simulink model "HighClearance_model"  (R2019b)
settings: configuration reference "configRef" (kept outside this file)
undefined symbols (not defined in the file): baseClearance, calSTEP1_e, calSTEP2_e, calSTEP3_e, calSTEP4_e, calTolMultiplier, errorMinSpd, heightCalibrating_e, heightDiffTolerance, heightDown_e, heightError_e, heightMovingDown_e, heightMovingUp_e, heightUnknown_e, heightUp_e, IOD_OK, IOD_Open, IOD_ScGnd, maxMedianWheelAngle, maxTransitionMachineSpd, minTransitionMachineSpd, positionSensor_tblData, positionSensorFL_BrkPnts, positionSensorFR_BrkPnts, positionSensorRL_BrkPnts, positionSensorRR_BrkPnts, step_time, trackWidthMax, trackWidthMin, trackWidthTolerance, twoWheelSteer
libraries: HighClearance_library x129, simulink x25
(part 3 of 3)

== stateflow chart HighClearance_model/Arbitration/TargetStateArbitration ==
  state states
    en,du: lowerOkay = ( okayToLower() && !disableLower() );
    raiseOkay = ( okayToRaise() && !disableRiase() );
    state out = leaveActiveState [function]
      (default) -> (junction 1676)
      (junction 1685) -> (junction 1686) [order 1] : [prevTargetState == heightMovingDown_e]
      (junction 1676) -> (junction 1685) [order 1] : [hasChangedTo(stopBtn,1)]
      (junction 1676) -> (junction 1696) [order 2]
      (junction 1685) -> (junction 1687) [order 2]
      (junction 1686) -> (junction 1690)
      (junction 1687) -> (junction 1690) : [prevTargetState == heightMovingUp_e]
      (junction 1690) -> (junction 1698)
      (junction 1696) -> (junction 1698) [order 1] : [manualOverride != 0]
      (junction 1696) -> (junction 1701) [order 2]
      (junction 1698) -> (junction 1700)
      (junction 1701) -> (junction 1700) [order 1] : [!calOkay()]
      (junction 1701) -> (junction 1711) [order 2]
      (junction 1700) -> (junction 1712)
      (junction 1711) -> (junction 1705) [order 1] : [prevTargetState == heightMovingDown_e]
      (junction 1705) -> (junction 1712) : [disableLower()]
      (junction 1711) -> (junction 1713) [order 2]
      (junction 1712) -> (junction 1714)
      (junction 1713) -> (junction 1706) [order 1] : [prevTargetState == heightMovingUp_e]
      (junction 1706) -> (junction 1714) : [disableRiase()]
      (junction 1713) -> (junction 1716) [order 2]
      (junction 1714) -> (junction 1717)
      (junction 1716) -> (junction 1717) [order 1] : [noMovementErr()]
      (junction 1716) -> (junction 1742) [order 2]
      (junction 1717) -> (junction 1734)
      (junction 1742) -> (junction 1733) [order 1] : [hasChangedTo(downBtn,1)]
      (junction 1733) -> (junction 1734) : [targetStateDown()]
      (junction 1742) -> (junction 1744) [order 2]
      (junction 1734) -> (junction 1738)
      (junction 1737) -> (junction 1738) : [targetStateUp()]
      (junction 1744) -> (junction 1737) [order 1] : [hasChangedTo(upBtn,1)]
      (junction 1744) -> (junction 1725) [order 2]
      (junction 1738) -> (junction 1728)
      (junction 1728) -> (junction 1730) : {out = true}
      (junction 1730) -> (junction 1723)
      (junction 1725) -> (junction 1723) : {out = false}
    state clearWarnings [function]
      (default) -> (junction 687) : {activeWarnings.trackWidth = 0;
          | activeWarnings.speed = 0;
          | activeWarnings.guide = 0;
          | activeWarnings.was = 0;
          | activeWarnings.fws = 0;
          | activeWarnings.fieldRoad = 0;
          | activeWarnings.cal = 0;
          | activeWarnings.parkBrake = 0;}
    state upWarnings [function]
      (default) -> (junction 973) : {activeWarnings.trackWidth = !trackWidthOkay();
          | activeWarnings.speed = !speedOkay();
          | activeWarnings.guide = 0;
          | activeWarnings.was = !wasOkay();
          | activeWarnings.fws = 0;
          | activeWarnings.fieldRoad = !fieldModeActive;
          | activeWarnings.cal = !calOkay();
          | activeWarnings.parkBrake = 0;}
    state downWarnings [function]
      (default) -> (junction 976) : {activeWarnings.trackWidth = !trackWidthOkay();
          | activeWarnings.speed = !speedOkay();
          | activeWarnings.guide = 0;
          | activeWarnings.was = !wasOkay();
          | activeWarnings.fws = 0;
          | activeWarnings.fieldRoad = !fieldModeActive;
          | activeWarnings.cal = !calOkay();
          | activeWarnings.parkBrake = !parkBrakeOkay();}
    state doNothing
      en:
      targetState = heightUnknown_e;
      clearWarnings();
      mfaLeds.downBtn = 0;
      mfaLeds.upBtn = 0;
    state active
      en: clearWarnings();
      (history)
      state paused
        en:
        targetState = heightUnknown_e;
      state wait
        en:
        clearWarnings();
      state out = pauseTransition [function]
        (default) -> (junction 927)
        (junction 927) -> (junction 981) [order 1] : [targetState == heightMovingUp_e]
        (junction 981) -> (junction 931) : [!okayToRaise()]
        (junction 931) -> (junction 984) : {upWarnings()}
        (junction 927) -> (junction 933) [order 2]
        (junction 984) -> (junction 937)
        (junction 986) -> (junction 988) : [!okayToLower()]
        (junction 988) -> (junction 937) : {downWarnings()}
        (junction 933) -> (junction 986) [order 1] : [targetState == heightMovingDown_e]
        (junction 933) -> (junction 991) [order 2]
        (junction 937) -> (junction 938) : {out = true}
        (junction 991) -> (junction 932)
        (junction 932) -> (junction 938) : {out = false}
      state out = restartTransition [function]
        (default) -> (junction 1027)
        (junction 1027) -> (junction 1028) [order 1] : [prevTargetState == heightMovingUp_e]
        (junction 1028) -> (junction 1029) : [okayToRaise()]
        (junction 1027) -> (junction 1030) [order 2]
        (junction 1029) -> (junction 1032)
        (junction 1030) -> (junction 1031) [order 1] : [prevTargetState == heightMovingDown_e]
        (junction 1031) -> (junction 1032) : [okayToLower()]
        (junction 1030) -> (junction 1034) [order 2]
        (junction 1032) -> (junction 1035) : {out = true}
        (junction 1034) -> (junction 1035) : {out = false}
      state transitioning
        (history)
        state up
          en:
          targetState = heightMovingUp_e;
          prevTargetState = heightMovingUp_e;
          mfaLeds.upBtn = 2;
          mfaLeds.downBtn = 0;
        state down
          en:
          targetState = heightMovingDown_e;
          prevTargetState = heightMovingDown_e;
          mfaLeds.upBtn = 0;
          mfaLeds.downBtn = 2;
      state holdUp
        en:
        targetState = heightUp_e;
        prevTargetState = heightUp_e;
        mfaLeds.upBtn = 1;
        mfaLeds.downBtn = 0;
      state holdDown
        en:
        targetState = heightDown_e;
        prevTargetState = heightDown_e;
        mfaLeds.upBtn = 0;
        mfaLeds.downBtn = 1;
      paused -> wait : after(20,msec)
      transitioning -> paused : [pauseTransition()]
      wait -> (junction 1563) : [restartTransition()]
      (junction 1563) -> transitioning
      up -> holdUp : [actualState == heightUp_e]
      down -> holdDown : [actualState == heightDown_e]
    state updateWarningsUp
      en: upWarnings();
    state updateWarningsDown
      en: downWarnings();
    state waitForEngineRunning
      en:
      targetState = heightUnknown_e;
      mfaLeds.downBtn = 0;
      mfaLeds.upBtn = 0;
    state out = okayToLower [function]
      (junction 1653) -> (junction 1652) : [trackWidthOkay()]
      (junction 741) -> (junction 1653) [order 2]
      (junction 1652) -> (junction 742)
      (default) -> (junction 737)
      (junction 739) -> (junction 740)
      (junction 737) -> (junction 1545) [order 1] : [parkBrakeOkay()]
      (junction 1545) -> (junction 738) : [speedOkay()]
      (junction 738) -> (junction 739) : [wasOkay()]
      (junction 740) -> (junction 741) : [fieldModeActive]
      (junction 741) -> (junction 742) [order 1] : [trackWidthError()]
      (junction 737) -> (junction 743) [order 2]
      (junction 742) -> (junction 748) : {out = true}
      (junction 743) -> (junction 748) : {out = false}
    state out = disableLower [function]
      (default) -> (junction 1251)
      (junction 1251) -> (junction 1400) [order 1] : [prevTargetState == heightMovingDown_e]
      (junction 1400) -> (junction 1252) : [!mfaAlive]
      (junction 1251) -> (junction 1415) [order 2]
      (junction 1252) -> (junction 1407)
      (junction 1415) -> (junction 1265)
      (junction 1407) -> (junction 1266) : {out = true}
      (junction 1265) -> (junction 1266) : {out = false}
    state out = trackWidthError [function]
      (default) -> (junction 834)
      (junction 834) -> (junction 835) [order 1] : [trackWidth.FrontLeft <= 0]
      (junction 834) -> (junction 836) [order 2]
      (junction 835) -> (junction 837)
      (junction 836) -> (junction 837) [order 1] : [trackWidth.FrontRight <= 0]
      (junction 836) -> (junction 838) [order 2]
      (junction 837) -> (junction 839)
      (junction 838) -> (junction 839) [order 1] : [trackWidth.RearLeft <= 0]
      (junction 838) -> (junction 840) [order 2]
      (junction 839) -> (junction 841)
      (junction 840) -> (junction 841) [order 1] : [trackWidth.RearRight <= 0]
      (junction 840) -> (junction 842) [order 2] : {out = false}
      (junction 841) -> (junction 843) : {out = true}
      (junction 843) -> (junction 842)
    state out = trackRngCheck(width) [function]
      (default) -> (junction 782)
      (junction 782) -> (junction 783) [order 1] : [!trackWidthError()]
      (junction 783) -> (junction 784) : [width >= (trackWidthMin - trackWidthTolerance)]
      (junction 782) -> (junction 785) [order 2] : {out = false}
      (junction 784) -> (junction 786) : [width <= (trackWidthMax + trackWidthTolerance)]
      (junction 786) -> (junction 785) : {out = true}
    state out = requireSpeed [function]
      (default) -> (junction 718)
      (junction 718) -> (junction 719) [commented out] : [trackWidthError()]
      (junction 719) -> (junction 721) [commented out]
      (junction 718) -> (junction 720)
      (junction 720) -> (junction 721) [commented out] : [actualState == heightError_e]
      (junction 720) -> (junction 1581)
      (junction 721) -> (junction 1579) [commented out]
      (junction 1581) -> (junction 1579) [commented out] : [!calOkay()]
      (junction 1581) -> (junction 1107)
      (junction 1579) -> (junction 1109) [commented out]
      (junction 1107) -> (junction 1109) [commented out] : [(cylCoilDiags.retract.FrontLeft & IOD_Open) == IOD_Open]
      (junction 1107) -> (junction 1113)
      (junction 1109) -> (junction 1114) [commented out]
      (junction 1113) -> (junction 1114) [commented out] : [(cylCoilDiags.retract.FrontRight & IOD_Open) == IOD_Open]
      (junction 1114) -> (junction 1122) [commented out]
      (junction 1113) -> (junction 1121)
      (junction 1121) -> (junction 1122) [commented out] : [(cylCoilDiags.retract.RearLeft & IOD_Open) == IOD_Open]
      (junction 1122) -> (junction 1125) [commented out]
      (junction 1121) -> (junction 1124)
      (junction 1124) -> (junction 1125) [commented out] : [(cylCoilDiags.retract.RearRight & IOD_Open) == IOD_Open]
      (junction 1125) -> (junction 722) [commented out]
      (junction 1124) -> (junction 1180)
      (junction 1180) -> (junction 722) [commented out] : [trackCylError()]
      (junction 1180) -> (junction 723)
      (junction 722) -> (junction 724) [commented out] : {out = true}
      (junction 723) -> (junction 724) : {out = false}
    state out = calOkay [function]
      (default) -> (junction 768)
      (junction 768) -> (junction 769) [order 1] : [actualState != heightCalibrating_e]
      (junction 768) -> (junction 771) [order 2] : {out = false}
      (junction 769) -> (junction 770) : [posCalOkay]
      (junction 770) -> (junction 772) : {out = true}
      (junction 771) -> (junction 772)
    state out = wasOkay [function]
      note: %No Front wheel angle requirement
      (default) -> (junction 795)
      (junction 795) -> (junction 1667) [order 1] : [1==1]
      (junction 795) -> (junction 1663) [order 2] : [abs(medianWheelAngle) > maxMedianWheelAngle]
      (junction 1667) -> (junction 1668)
      (junction 795) -> (junction 1665) [order 3] : [!prevWasOkayOut]
      (junction 1663) -> (junction 798) : {out = false}
      (junction 1665) -> (junction 796) : [abs(medianWheelAngle) <= (maxMedianWheelAngle - 2)]
      (junction 1668) -> (junction 796)
      (junction 796) -> (junction 798) : {out = true}
      (junction 798) -> (junction 1660) : {prevWasOkayOut = out}
    state out = targetStateSelected [function]
      (default) -> (junction 1068)
      (junction 1068) -> (junction 1069) [order 1] : [targetState == heightDown_e]
      (junction 1068) -> (junction 1070) [order 2]
      (junction 1069) -> (junction 1071)
      (junction 1070) -> (junction 1071) [order 1] : [targetState == heightUp_e]
      (junction 1070) -> (junction 1085) [order 2]
      (junction 1071) -> (junction 1091)
      (junction 1085) -> (junction 1091) [order 1] : [targetState == heightMovingUp_e]
      (junction 1085) -> (junction 1092) [order 2]
      (junction 1091) -> (junction 1087)
      (junction 1092) -> (junction 1087) [order 1] : [targetState == heightMovingDown_e]
      (junction 1092) -> (junction 1073) [order 2]
      (junction 1087) -> (junction 1074) : {out = true}
      (junction 1073) -> (junction 1074) : {out = false}
    state out = okayToRaise [function]
      (default) -> (junction 894)
      (junction 1304) -> (junction 1298)
      (junction 894) -> (junction 1547) [order 1]
      (junction 1547) -> (junction 1247)
      (junction 1247) -> (junction 1195) : [trackWidthOkay()]
      (junction 1195) -> (junction 1305) : [speedOkay()]
      (junction 1305) -> (junction 1304) : [wasOkay()]
      (junction 1298) -> (junction 896) : [fieldModeActive]
      (junction 894) -> (junction 897) [order 2]
      (junction 896) -> (junction 899) : {out = true}
      (junction 897) -> (junction 899) : {out = false}
    state out = disableRiase [function]
      (default) -> (junction 1420)
      (junction 1420) -> (junction 1448) [order 1] : [prevTargetState == heightMovingUp_e]
      (junction 1448) -> (junction 1635) [order 1] : [!mfaAlive]
      (junction 1420) -> (junction 1423) [order 2]
      (junction 1448) -> (junction 1421) [order 2]
      (junction 1635) -> (junction 1422)
      (junction 1423) -> (junction 1421) [order 1] : [prevTargetState == heightDown_e]
      (junction 1421) -> (junction 1422) [order 1] : [trackWidthError()]
      (junction 1423) -> (junction 1426) [order 2]
      (junction 1421) -> (junction 1424) [order 2]
      (junction 1422) -> (junction 1425)
      (junction 1424) -> (junction 1425) [order 1] : [trackCylError()]
      (junction 1424) -> (junction 1647) [order 2]
      (junction 1425) -> (junction 1650)
      (junction 1647) -> (junction 1650) [order 1] : [!dwnBtnOk]
      (junction 1647) -> (junction 1457) [order 2]
      (junction 1650) -> (junction 1446)
      (junction 1457) -> (junction 1446) [order 1] : [actualState == heightError_e]
      (junction 1457) -> (junction 1464) [order 2]
      (junction 1446) -> (junction 1466)
      (junction 1464) -> (junction 1466) [order 1] : [cylCoilDiags.extend.FrontLeft != IOD_OK]
      (junction 1464) -> (junction 1470) [order 2]
      (junction 1466) -> (junction 1468)
      (junction 1470) -> (junction 1468) [order 1] : [cylCoilDiags.extend.FrontRight != IOD_OK]
      (junction 1470) -> (junction 1473) [order 2]
      (junction 1468) -> (junction 1471)
      (junction 1473) -> (junction 1471) [order 1] : [cylCoilDiags.extend.RearLeft != IOD_OK]
      (junction 1473) -> (junction 1476) [order 2]
      (junction 1471) -> (junction 1474)
      (junction 1476) -> (junction 1474) [order 1] : [cylCoilDiags.extend.RearRight != IOD_OK]
      (junction 1476) -> (junction 1495) [order 2]
      (junction 1474) -> (junction 1485)
      (junction 1495) -> (junction 1485) [order 1] : [cylCoilDiags.retract.FrontLeft != IOD_OK]
      (junction 1495) -> (junction 1489) [order 2]
      (junction 1485) -> (junction 1487)
      (junction 1489) -> (junction 1487) [order 1] : [cylCoilDiags.retract.FrontRight != IOD_OK]
      (junction 1489) -> (junction 1488) [order 2]
      (junction 1487) -> (junction 1484)
      (junction 1488) -> (junction 1484) [order 1] : [cylCoilDiags.retract.RearLeft != IOD_OK]
      (junction 1488) -> (junction 1498) [order 2]
      (junction 1484) -> (junction 1493)
      (junction 1498) -> (junction 1493) [order 1] : [cylCoilDiags.retract.RearRight != IOD_OK]
      (junction 1498) -> (junction 1452) [order 2]
      (junction 1493) -> (junction 1427) : {out = true}
      (junction 1426) -> (junction 1452)
      (junction 1452) -> (junction 1427) : {out = false}
    state out = trackCylError [function]
      (default) -> (junction 1136)
      (junction 1136) -> (junction 1137) [order 1] : [trackCylCoilDiags.extend.FrontLeft != IOD_OK]
      (junction 1136) -> (junction 1138) [order 2]
      (junction 1137) -> (junction 1139)
      (junction 1138) -> (junction 1139) [order 1] : [trackCylCoilDiags.extend.FrontRight != IOD_OK]
      (junction 1138) -> (junction 1140) [order 2]
      (junction 1139) -> (junction 1141)
      (junction 1140) -> (junction 1141) [order 1] : [trackCylCoilDiags.extend.RearLeft != IOD_OK]
      (junction 1140) -> (junction 1142) [order 2]
      (junction 1141) -> (junction 1143)
      (junction 1142) -> (junction 1143) [order 1] : [trackCylCoilDiags.extend.RearRight != IOD_OK]
      (junction 1142) -> (junction 1163) [order 2]
      (junction 1143) -> (junction 1167)
      (junction 1163) -> (junction 1167) [order 1] : [trackCylCoilDiags.retract.FrontLeft != IOD_OK]
      (junction 1163) -> (junction 1161) [order 2]
      (junction 1167) -> (junction 1160)
      (junction 1161) -> (junction 1160) [order 1] : [trackCylCoilDiags.retract.FrontRight != IOD_OK]
      (junction 1161) -> (junction 1162) [order 2]
      (junction 1160) -> (junction 1170)
      (junction 1162) -> (junction 1170) [order 1] : [trackCylCoilDiags.retract.RearLeft != IOD_OK]
      (junction 1162) -> (junction 1174) [order 2]
      (junction 1170) -> (junction 1173)
      (junction 1174) -> (junction 1173) [order 1] : [trackCylCoilDiags.retract.RearRight != IOD_OK]
      (junction 1174) -> (junction 1144) [order 2] : {out = false}
      (junction 1173) -> (junction 1145) : {out = true}
      (junction 1145) -> (junction 1144)
    state out = trackWidthOkay [function]
      (default) -> (junction 807)
      (junction 807) -> (junction 806) [order 2]
      (junction 806) -> (junction 808)
      (junction 807) -> (junction 809) [order 1] : [trackRngCheck(trackWidth.FrontLeft)]
      (junction 809) -> (junction 808) [order 2]
      (junction 808) -> (junction 810)
      (junction 809) -> (junction 811) [order 1] : [trackRngCheck(trackWidth.FrontRight)]
      (junction 811) -> (junction 810) [order 2]
      (junction 810) -> (junction 812)
      (junction 811) -> (junction 813) [order 1] : [trackRngCheck(trackWidth.RearLeft)]
      (junction 813) -> (junction 812) [order 2]
      (junction 812) -> (junction 815) : {out = false}
      (junction 813) -> (junction 814) [order 1] : [trackRngCheck(trackWidth.RearRight)]
      (junction 814) -> (junction 816) : {out = true}
      (junction 815) -> (junction 816)
    state out = speedOkay [function]
      (default) -> (junction 871)
      (junction 871) -> (junction 872) [order 1] : [requireSpeed()]
      (junction 872) -> (junction 873) : [machineSpeed > errorMinSpd]
      (junction 871) -> (junction 874) [order 2]
      (junction 873) -> (junction 875)
      (junction 874) -> (junction 875) [order 1] : [machineSpeed >= minTransitionMachineSpd]
      (junction 875) -> (junction 876) [order 1] : [machineSpeed <= maxTransitionMachineSpd]
      (junction 874) -> (junction 879) [order 2]
      (junction 875) -> (junction 877) [order 2]
      (junction 876) -> (junction 878) : {out = true}
      (junction 877) -> (junction 878) : {out = false}
      (junction 879) -> (junction 877)
    state out = targetStateDown [function]
      (default) -> (junction 1320)
      (junction 1320) -> (junction 1321) [order 1] : [targetState == heightDown_e]
      (junction 1320) -> (junction 1322) [order 2]
      (junction 1321) -> (junction 1323)
      (junction 1322) -> (junction 1323) [order 1] : [targetState == heightMovingDown_e]
      (junction 1322) -> (junction 1334) [order 2]
      (junction 1323) -> (junction 1335) : {out = true}
      (junction 1334) -> (junction 1335) : {out = false}
    state out = targetStateUp [function]
      (default) -> (junction 1361)
      (junction 1361) -> (junction 1362) [order 1] : [targetState == heightUp_e]
      (junction 1361) -> (junction 1363) [order 2]
      (junction 1362) -> (junction 1364)
      (junction 1363) -> (junction 1364) [order 1] : [targetState == heightMovingUp_e]
      (junction 1363) -> (junction 1375) [order 2]
      (junction 1364) -> (junction 1376) : {out = true}
      (junction 1375) -> (junction 1376) : {out = false}
    state out = noMovementErr [function]
      (default) -> (junction 1516)
      (junction 1516) -> (junction 1518) [order 1] : [legErrors.FrontLeft.noMovementErr]
      (junction 1516) -> (junction 1515) [order 2]
      (junction 1518) -> (junction 1520)
      (junction 1515) -> (junction 1520) [order 1] : [legErrors.FrontRight.noMovementErr]
      (junction 1515) -> (junction 1517) [order 2]
      (junction 1520) -> (junction 1522)
      (junction 1517) -> (junction 1522) [order 1] : [legErrors.RearLeft.noMovementErr]
      (junction 1517) -> (junction 1519) [order 2]
      (junction 1522) -> (junction 1523)
      (junction 1519) -> (junction 1523) [order 1] : [legErrors.RearRight.noMovementErr]
      (junction 1519) -> (junction 1524) [order 2] : {out = false}
      (junction 1523) -> (junction 1525) : {out = true}
      (junction 1524) -> (junction 1525)
    state out = parkBrakeOkay [function]
      (default) -> (junction 1551)
      (junction 1551) -> (junction 1552) [order 1] : [selectedGear != 251]
      (junction 1551) -> (junction 1553) [order 2] : {out = false}
      (junction 1552) -> (junction 1554) : {out = true}
      (junction 1554) -> (junction 1553)
    active -> doNothing [order 1] : [leaveActiveState()]
    (junction 705) -> doNothing [order 2]
    (junction 705) -> active [order 1] : [targetStateSelected()]
    updateWarningsUp -> (junction 705) : after(20,msec)
    (junction 1628) -> up : [!disableRiase()]
    (junction 1624) -> (junction 1628) [order 2] : [okayToRaise()]
    (junction 1569) -> holdUp
    (junction 1567) -> (junction 1569)
    (junction 267) -> updateWarningsUp [order 2]
    doNothing -> (junction 267) [order 1] : [hasChangedTo(upBtn,1)]
    (junction 267) -> (junction 1624) [order 1] : [calOkay()]
    (junction 1624) -> holdUp [order 1] : [actualState == heightUp_e]
    (junction 270) -> (junction 267)
    (junction 1197) -> (junction 270) : [targetStateDown()]
    active -> (junction 1197) [order 2] : [hasChangedTo(upBtn,1)]
    (junction 1199) -> (junction 282) : [targetStateUp()]
    active -> (junction 1199) [order 3] : [hasChangedTo(downBtn,1)]
    (junction 282) -> (junction 125)
    doNothing -> (junction 125) [order 2] : [hasChangedTo(downBtn,1)]
    (junction 125) -> (junction 1619) [order 1] : [calOkay()]
    (junction 1619) -> holdDown [order 1] : [actualState == heightDown_e]
    (junction 125) -> updateWarningsDown [order 2]
    (junction 1619) -> (junction 1630) [order 2] : [okayToLower() ]
    (junction 1630) -> down : [!disableLower()]
    updateWarningsDown -> (junction 702) : after(20,msec)
    (junction 1566) -> holdDown [order 1] : [actualState == heightDown_e]
    (junction 702) -> doNothing [order 2]
    (junction 702) -> active [order 1] : [targetStateSelected()]
    (junction 1575) -> doNothing
    (junction 1613) -> (junction 1575)
    (junction 1616) -> (junction 1613)
    (junction 1566) -> (junction 1616) [order 2]
    (junction 1609) -> (junction 1613) [order 2]
    (junction 1611) -> (junction 1616) [order 2]
    (junction 1572) -> (junction 1566) [order 2]
    waitForEngineRunning -> (junction 1609) : [engRunning]
    (junction 1609) -> (junction 1611) [order 1] : [fieldModeActive]
    (junction 1611) -> (junction 1572) [order 1] : [calOkay()]
    (junction 1572) -> (junction 1567) [order 1] : [actualState == heightUp_e]
    (default) -> waitForEngineRunning
  (default) -> states
  states -> states : [hasChangedTo(engRunning,0)]
  data: out function_output boolean; out function_output double; out function_output double; out function_output boolean; out function_output boolean; out function_output boolean; out function_output boolean; width function_input single; out function_output boolean; out function_output boolean; out function_output boolean; out function_output boolean; out function_output boolean; out function_output boolean; out function_output boolean; out function_output boolean; out function_output boolean; out function_output boolean; out function_output boolean; out function_output boolean; out function_output boolean; heightDown_e parameter; heightUp_e parameter; heightCalibrating_e parameter; heightError_e parameter; heightUnknown_e parameter; upBtn input; downBtn input; stopBtn input; mfaAlive input boolean; dwnBtnOk input boolean; targetState output uint8; twoWheelSteer parameter; maxMedianWheelAngle parameter; maxTransitionMachineSpd parameter; minTransitionMachineSpd parameter; activeWarnings output Bus: UserWarningBus; mfaLeds output Bus: MfaBus =0; trackWidthMin parameter; trackWidthMax parameter; engRunning input boolean; posCalOkay input; fieldModeActive input boolean; trackWidth input Bus: CylinderBus; machineSpeed input; medianWheelAngle input; cylCoilDiags input Bus: CoilStateBus; ccoEnableDiag input; trackCylCoilDiags input Bus: CoilStateBus; legErrors input Bus: ErrorsBus; selectedGear input; manualOverride input; actualState input; errorMinSpd parameter; prevTargetState local uint8; heightMovingDown_e parameter; heightMovingUp_e parameter; raiseOkay output boolean; lowerOkay output boolean; IOD_Open parameter; IOD_ScGnd parameter; IOD_OK parameter; prevWasOkayOut local boolean =0; trackWidthTolerance parameter

== stateflow chart HighClearance_model/Arbitration/ActualStateArbitration/actualMachineState ==
  state out = checkError [function]
    (default) -> (junction 412)
    (junction 412) -> (junction 415) [order 1] : [legState.FrontLeft == heightError_e]
    (junction 412) -> (junction 417) [order 2]
    (junction 415) -> (junction 427)
    (junction 417) -> (junction 427) [order 1] : [legState.FrontRight == heightError_e]
    (junction 417) -> (junction 419) [order 2]
    (junction 427) -> (junction 428)
    (junction 419) -> (junction 428) [order 1] : [legState.RearLeft == heightError_e]
    (junction 419) -> (junction 420) [order 2]
    (junction 428) -> (junction 433)
    (junction 420) -> (junction 433) [order 1] : [legState.RearRight == heightError_e]
    (junction 420) -> (junction 439) [order 2] : {out = 0}
    (junction 433) -> (junction 424) : {out = 1}
    (junction 424) -> (junction 439)
  state out = checkMovingUp [function]
    (default) -> (junction 457)
    (junction 457) -> (junction 458) [order 1] : [legState.FrontLeft == heightMovingUp_e]
    (junction 457) -> (junction 459) [order 2]
    (junction 458) -> (junction 460)
    (junction 459) -> (junction 460) [order 1] : [legState.FrontRight == heightMovingUp_e]
    (junction 459) -> (junction 461) [order 2]
    (junction 460) -> (junction 462)
    (junction 461) -> (junction 462) [order 1] : [legState.RearLeft == heightMovingUp_e]
    (junction 461) -> (junction 463) [order 2]
    (junction 462) -> (junction 464)
    (junction 463) -> (junction 464) [order 1] : [legState.RearRight == heightMovingUp_e]
    (junction 463) -> (junction 465) [order 2] : {out = 0}
    (junction 464) -> (junction 466) : {out = 1}
    (junction 466) -> (junction 465)
  state out = checkMovingDown [function]
    (default) -> (junction 483)
    (junction 483) -> (junction 484) [order 1] : [legState.FrontLeft == heightMovingDown_e]
    (junction 483) -> (junction 485) [order 2]
    (junction 484) -> (junction 486)
    (junction 485) -> (junction 486) [order 1] : [legState.FrontRight == heightMovingDown_e]
    (junction 485) -> (junction 487) [order 2]
    (junction 486) -> (junction 488)
    (junction 487) -> (junction 488) [order 1] : [legState.RearLeft == heightMovingDown_e]
    (junction 487) -> (junction 489) [order 2]
    (junction 488) -> (junction 490)
    (junction 489) -> (junction 490) [order 1] : [legState.RearRight == heightMovingDown_e]
    (junction 489) -> (junction 491) [order 2] : {out = 0}
    (junction 490) -> (junction 492) : {out = 1}
    (junction 492) -> (junction 491)
  state out = checkCalibrating [function]
    (default) -> (junction 614)
    (junction 614) -> (junction 633) [order 1] : [calibrationActive]
    (junction 614) -> (junction 634) [order 2] : {out = false}
    (junction 633) -> (junction 637) : {out = true}
    (junction 637) -> (junction 634)
  state out = checkUnknown [function] [commented out]
    (default) -> (junction 553) [commented out]
    (junction 553) -> (junction 554) [commented out] : [checkMovingUp()]
    (junction 553) -> (junction 558) [commented out] : {out = 0}
    (junction 554) -> (junction 557) [commented out] : [checkMovingDown()]
    (junction 557) -> (junction 559) [commented out] : {out = 1}
    (junction 559) -> (junction 558) [commented out]
  state out = checkUp [function]
    (default) -> (junction 509)
    (junction 509) -> (junction 510) [order 1] : [legState.FrontLeft == heightUp_e]
    (junction 509) -> (junction 517) [order 2] : {out = 0}
    (junction 510) -> (junction 512) : [legState.FrontRight == heightUp_e]
    (junction 512) -> (junction 514) : [legState.RearLeft == heightUp_e]
    (junction 514) -> (junction 516) : [legState.RearRight == heightUp_e]
    (junction 516) -> (junction 518) : {out = 1}
    (junction 518) -> (junction 517)
  state out = checkDown [function]
    (default) -> (junction 535)
    (junction 535) -> (junction 536) [order 1] : [legState.FrontLeft == heightDown_e]
    (junction 535) -> (junction 540) [order 2] : {out = 0}
    (junction 536) -> (junction 537) : [legState.FrontRight == heightDown_e]
    (junction 537) -> (junction 538) : [legState.RearLeft == heightDown_e]
    (junction 538) -> (junction 539) : [legState.RearRight == heightDown_e]
    (junction 539) -> (junction 541) : {out = 1}
    (junction 541) -> (junction 540)
  state states
    state error
      en:
      machineState = heightError_e;
    state calibrating
      en: machineState = heightCalibrating_e;
    state down
      en:
      machineState = heightDown_e;
    state up
      en:
      machineState = heightUp_e;
    state movingDown
      en:
      machineState = heightMovingDown_e;
    state movingUp
      en:
      machineState = heightMovingUp_e;
    state unKnown
      en:
      machineState = heightUnknown_e;
  (default) -> (junction 588)
  (junction 588) -> (junction 569)
  (junction 569) -> (junction 627) [order 2]
  (junction 627) -> (junction 594) [order 2]
  (junction 594) -> (junction 597) [order 2]
  (junction 597) -> (junction 600) [order 2]
  (junction 600) -> (junction 603) [order 2]
  (junction 603) -> (junction 604) [order 2]
  states -> (junction 588) : after(step_time,msec)
  (junction 569) -> error [order 1] : [checkError()]
  (junction 627) -> calibrating [order 1] : [checkCalibrating()]
  (junction 594) -> down [order 1] : [checkDown()]
  (junction 597) -> up [order 1] : [checkUp()]
  (junction 600) -> movingDown [order 1] : [checkMovingDown()]
  (junction 603) -> movingUp [order 1] : [checkMovingUp()]
  (junction 604) -> unKnown
  data: out function_output boolean; out function_output boolean; out function_output boolean; out function_output boolean; out function_output boolean; out function_output boolean; out function_output boolean; machineState output uint8; heightDown_e parameter; heightUp_e parameter; heightMovingUp_e parameter; heightMovingDown_e parameter; heightCalibrating_e parameter; heightError_e parameter; heightUnknown_e parameter; legState input Bus: StateBus; calibrationActive input; step_time parameter

== stateflow chart HighClearance_model/Calibration/controlLogic/calStateConverstion/calState2TargetState ==
  state states
    state stop
      en: targetState = heightUnknown_e;
    state Down
      en: targetState = heightDown_e;
    state Up
      en: targetState = heightUp_e;
    (default) -> (junction 15)
    (junction 15) -> stop [order 3]
    (junction 15) -> Down [order 1] : [calState == calSTEP1_e ||...
        | calState == calSTEP2_e]
    (junction 15) -> Up [order 2] : [calState == calSTEP3_e ||...
        | calState == calSTEP4_e]
  states -> states : [hasChanged(calState)]
  (default) -> states
  data: calState input; targetState output uint8; calSTEP1_e parameter; calSTEP2_e parameter; calSTEP3_e parameter; calSTEP4_e parameter; heightUp_e parameter; heightDown_e parameter; heightUnknown_e parameter

== stateflow chart HighClearance_model/Control/manualOverrides/manualOverrides ==
  state setIO [function]
    (default) -> (junction 17)
    (junction 17) -> (junction 19) [order 2] : [override == 0xDD01]
    (junction 17) -> (junction 18) [order 1] : [override == 0xAA01]
    (junction 19) -> (junction 72) : {pwm.retract.FrontLeft = false}
    (junction 18) -> (junction 36) : {pwm.retract.FrontLeft = bangBang_maxOut}
    (junction 72) -> (junction 74)
    (junction 17) -> (junction 61) [order 3]
    (junction 36) -> (junction 64)
    (junction 73) -> (junction 74) : {pwm.extend.FrontLeft = false}
    (junction 62) -> (junction 64) : {pwm.extend.FrontLeft = bangBang_maxOut}
    (junction 61) -> (junction 73) [order 2] : [override == 0xDD11]
    (junction 61) -> (junction 62) [order 1] : [override == 0xAA11]
    (junction 74) -> (junction 93)
    (junction 61) -> (junction 83) [order 3]
    (junction 64) -> (junction 79)
    (junction 83) -> (junction 81) [order 2] : [override == 0xDD02]
    (junction 83) -> (junction 80) [order 1] : [override == 0xAA02]
    (junction 81) -> (junction 93) : {pwm.retract.FrontRight = false}
    (junction 80) -> (junction 79) : {pwm.retract.FrontRight = bangBang_maxOut}
    (junction 93) -> (junction 91)
    (junction 83) -> (junction 94) [order 3]
    (junction 79) -> (junction 90)
    (junction 87) -> (junction 91) : {pwm.extend.FrontRight = false}
    (junction 95) -> (junction 90) : {pwm.extend.FrontRight = bangBang_maxOut}
    (junction 94) -> (junction 87) [order 2] : [override == 0xDD12]
    (junction 94) -> (junction 95) [order 1] : [override == 0xAA12]
    (junction 91) -> (junction 176)
    (junction 94) -> (junction 187) [order 3]
    (junction 90) -> (junction 159)
    (junction 187) -> (junction 160) [order 2] : [override == 0xDD03]
    (junction 187) -> (junction 161) [order 1] : [override == 0xAA03]
    (junction 160) -> (junction 176) : {pwm.retract.RearLeft = false}
    (junction 161) -> (junction 159) : {pwm.retract.RearLeft = bangBang_maxOut}
    (junction 176) -> (junction 175)
    (junction 187) -> (junction 156) [order 3]
    (junction 159) -> (junction 180)
    (junction 173) -> (junction 175) : {pwm.extend.RearLeft = false}
    (junction 168) -> (junction 180) : {pwm.extend.RearLeft = bangBang_maxOut}
    (junction 156) -> (junction 173) [order 2] : [override == 0xDD13]
    (junction 156) -> (junction 168) [order 1] : [override == 0xAA13]
    (junction 175) -> (junction 152)
    (junction 156) -> (junction 171) [order 3]
    (junction 180) -> (junction 166)
    (junction 165) -> (junction 152) : {pwm.retract.RearRight = false}
    (junction 178) -> (junction 166) : {pwm.retract.RearRight = bangBang_maxOut}
    (junction 171) -> (junction 165) [order 2] : [override == 0xDD04]
    (junction 171) -> (junction 178) [order 1] : [override == 0xAA04]
    (junction 152) -> (junction 150)
    (junction 171) -> (junction 169) [order 3]
    (junction 166) -> (junction 183)
    (junction 155) -> (junction 150) : {pwm.extend.RearRight = false}
    (junction 151) -> (junction 183) : {pwm.extend.RearRight = bangBang_maxOut}
    (junction 169) -> (junction 155) [order 2] : [override == 0xDD14]
    (junction 169) -> (junction 151) [order 1] : [override == 0xAA14]
    (junction 150) -> (junction 69)
    (junction 169) -> (junction 23) [order 3]
    (junction 183) -> (junction 67)
    (junction 69) -> (junction 23)
    (junction 67) -> (junction 23)
  state normal
    en: overrideEnabled = false;
  state overRided
    en: overrideEnabled = true;
    setIO();
  overRided -> overRided [order 2] : [hasChanged(override)]
  (default) -> normal
  normal -> overRided : [override != 0]
  overRided -> normal [order 1] : [override == 0]
  data: pwm output Bus: CoilBus; overrideEnabled output boolean; override input uint16; bangBang_maxOut parameter

== stateflow chart HighClearance_model/Arbitration/ladderExtendLogic ==
  state retract
    en:
    extendLadder = false;
  state extend
    en:
    extendLadder = true;
  state out = extendOkay [function]
    (default) -> (junction 15)
    (junction 15) -> (junction 19) [order 1] : [selectedGear == 251]
    (junction 19) -> (junction 17) : [machineState == heightUp_e]
    (junction 15) -> (junction 23) [order 2]
    (junction 17) -> (junction 22) : {out = true}
    (junction 23) -> (junction 22) : {out = false}
  (default) -> (junction 7)
  (junction 7) -> retract [order 2]
  (junction 7) -> extend [order 1] : [extendOkay()]
  extend -> retract : [!extendOkay()]
  retract -> extend : [extendOkay()]
  data: out function_output boolean; selectedGear input; machineState input; extendLadder output boolean; heightUp_e parameter

== stateflow chart HighClearance_model/Control/legEnablesLogic/legEnable__ ==
  state out = trackWidthInTolerance [function]
    (default) -> (junction 35)
    (junction 35) -> (junction 40) [order 1] : [(targetTrackPos - actualTrackPos) <= trackWidthTolerance]
    (junction 35) -> (junction 42) [order 2] : {out = false}
    (junction 40) -> (junction 41) : [(actualTrackPos - targetTrackPos) <= trackWidthTolerance]
    (junction 41) -> (junction 42) : {out = true}
  state out = heightInTolerance [function]
    (junction 106) -> (junction 108)
    (junction 117) -> (junction 119)
    (junction 124) -> (junction 128)
    (junction 71) -> (junction 106) [order 1] : [legHeightRef1 == 0]
    (junction 108) -> (junction 122)
    (junction 77) -> (junction 117) [order 1] : [legHeightRef2 == 0]
    (junction 119) -> (junction 125)
    (junction 80) -> (junction 124) [order 1] : [legHeightRef3 == 0]
    (junction 128) -> (junction 81)
    (junction 77) -> (junction 125) [order 2] : [( legHeightSubject - legHeightRef2 ) <= tolerance]
    (junction 80) -> (junction 81) [order 2] : [( legHeightSubject - legHeightRef3 ) <= tolerance]
    (junction 125) -> (junction 80)
    (junction 122) -> (junction 77)
    (junction 71) -> (junction 122) [order 2] : [( legHeightSubject - legHeightRef1 ) <= tolerance]
    (junction 69) -> (junction 71) [order 1] : [targetState == heightUp_e ||...
        | targetState == heightMovingUp_e]
    (junction 77) -> (junction 111) [order 3]
    (junction 80) -> (junction 114) [order 3]
    (junction 81) -> (junction 75) : {out = true}
    (default) -> (junction 69)
    (junction 69) -> (junction 111) [order 3]
    (junction 111) -> (junction 114)
    (junction 114) -> (junction 75) : {out = false}
    (junction 69) -> (junction 91) [order 2] : [targetState == heightDown_e ||...
        | targetState == heightMovingDown_e]
    (junction 86) -> (junction 111) [order 3]
    (junction 88) -> (junction 114) [order 3]
    (junction 87) -> (junction 75) : {out = true}
    (junction 131) -> (junction 86)
    (junction 132) -> (junction 88)
    (junction 91) -> (junction 131) [order 1] : [( legHeightRef1 - legHeightSubject ) <= tolerance]
    (junction 86) -> (junction 132) [order 2] : [( legHeightRef2 - legHeightSubject ) <= tolerance]
    (junction 88) -> (junction 87) [order 2] : [( legHeightRef3 - legHeightSubject ) <= tolerance]
    (junction 91) -> (junction 140) [order 2] : [legHeightRef1 == 0]
    (junction 142) -> (junction 131)
    (junction 86) -> (junction 146) [order 1] : [legHeightRef2 == 0]
    (junction 147) -> (junction 132)
    (junction 88) -> (junction 151) [order 1] : [legHeightRef3 == 0]
    (junction 153) -> (junction 87)
    (junction 140) -> (junction 142)
    (junction 146) -> (junction 147)
    (junction 151) -> (junction 153)
  state disabled
    en: enable = false;
    state transitioning
      state okay
      state badTrack
        state wait
        state warning
          en: warningTrack = 1;
          ex: warningTrack = 0;
        state clear
        (default) -> disabled.transitioning.badTrack.wait
        disabled.transitioning.badTrack.wait -> disabled.transitioning.badTrack.warning : after(5,sec)
        disabled.transitioning.badTrack.warning -> disabled.transitioning.badTrack.clear
      state badHeight
        state warning
          en: warningHeight = 1;
          ex: warningHeight = 0;
        state wait
        state clear
        (default) -> disabled.transitioning.badHeight.wait
        disabled.transitioning.badHeight.wait -> disabled.transitioning.badHeight.warning : after(5,sec)
        disabled.transitioning.badHeight.warning -> disabled.transitioning.badHeight.clear
      (default) -> okay
      okay -> badTrack [order 1] : [!trackWidthInTolerance()]
      badTrack -> okay : [trackWidthInTolerance]
      okay -> badHeight [order 2] : [!heightInTolerance()]
      badHeight -> okay : [heightInTolerance()]
    state NotTransitioning
      en:
      warningTrack = 0;
      warningHeight = 0;
    (default) -> NotTransitioning
    (junction 173) -> transitioning : [targetState == heightMovingUp_e]
    (junction 172) -> (junction 173) [order 1]
    NotTransitioning -> (junction 172) : [legHeightSubject != 0]
    (junction 172) -> transitioning [order 2] : [targetState == heightMovingDown_e]
    transitioning -> NotTransitioning [order 1] : [legHeightSubject == 0]
    (junction 183) -> NotTransitioning : [targetState == heightMovingUp_e]
    transitioning -> (junction 183) [order 2] : [targetState != heightMovingDown_e]
  state enabled
    en: enable = true;
  (default) -> disabled
  disabled -> (junction 162) : [legHeightSubject != 0]
  (junction 162) -> (junction 207) : [legState != heightUp_e]
  (junction 207) -> (junction 38) : [trackWidthInTolerance()]
  (junction 38) -> enabled : [heightInTolerance()]
  enabled -> disabled [order 1] : [legHeightSubject == 0]
  enabled -> disabled [order 2] : [legState == heightUp_e]
  enabled -> disabled [order 3] : [!heightInTolerance()]
  enabled -> disabled [order 4] : [!trackWidthInTolerance()]
  data: out function_output boolean; out function_output boolean; targetState input; actualState input; legState input; enable output uint8; targetTrackPos input; actualTrackPos input; legHeightSubject input; legHeightRef1 input; legHeightRef2 input; legHeightRef3 input; heightDown_e parameter; heightUp_e parameter; heightMovingUp_e parameter; heightMovingDown_e parameter; heightCalibrating_e parameter; heightError_e parameter; heightUnknown_e parameter; trackWidthTolerance parameter; heightDiffTolerance parameter; tolerance input; warningTrack output uint8; warningHeight output uint8

== stateflow chart HighClearance_model/Arbitration/latch ==
  state isAlive
    en:
    alive = true;
  state notAlive
    en:
    alive = false;
  note: startup delay
  (default) -> isAlive
  isAlive -> (junction 7) : after(30,sec)
  (junction 7) -> notAlive : [!status]
  data: status input uint8; alive output boolean

== stateflow chart HighClearance_model/Arbitration/latch1 ==
  state okay
    en:
    dwnBtnOk = true;
  state notOkay
    en:
    dwnBtnOk = false;
  note: startup delay
  (default) -> okay
  okay -> (junction 7) : after(30,sec)
  (junction 7) -> notOkay : [diag]
  data: diag input; dwnBtnOk output boolean
